simulink model "cantoni_combined_matrices"  (R2019a)
settings: Solver=FixedStepDiscrete  StartTime=0.0  StopTime=1400  FixedStep=h  RelTol=1e-3
values from neighbouring files (symbols this model uses):
  comb_contr = ss(Ac, Bc, Cc, Dc, h)    [cantoni_LMI.m]
  comb_plant_disc = c2d(comb_plant_cont,h,'zoh')    [cantoni_LMI.m]
  h = 1    [cantoni_LMI.m]    (also in distributed_workspace.mat; model_hil.m = 0.00208333333333)
settings Model: Creator=Jacob  LastModifiedBy=Jacob

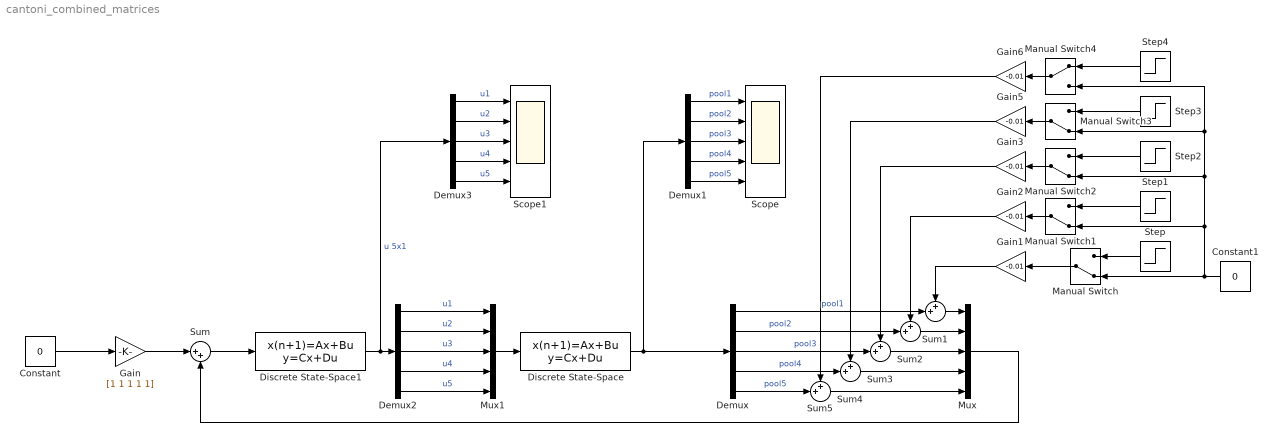
== system cantoni_combined_matrices ==
  Constant : Constant  Value=0
  Constant1 : Constant  Value=0
  Demux{,1..3} (4 alike) : Demux  Outputs=5
  Discrete State-Space : DiscreteStateSpace  A=comb_plant_disc.A  B=comb_plant_disc.B  C=comb_plant_disc.C  D=comb_plant_disc.D  SampleTime=h
  Discrete State-Space1 : DiscreteStateSpace  A=comb_contr.A  B=comb_contr.B  C=comb_contr.C  D=comb_contr.D  SampleTime=h
  Gain : Gain  Gain=[1 1 1 1 1]
  Gain{1..3,5..6} (5 alike) : Gain  Gain=-0.01
  Manual Switch{,1..3} (4 alike) : ManualSwitch  CurrentSetting=0
  Manual Switch4 : ManualSwitch
  Mux : Mux  Inputs=5
  Mux1 : Mux  Inputs=5
  Scope : Scope  NumInputPorts=5
  Scope1 : Scope  NumInputPorts=5
  Step{,1..4} (5 alike) : Step  Time=50  SampleTime=0
  Sum : Sum  Inputs=|++
  Sum{1..5} (5 alike) : Sum  Inputs=++|
  wires:
  Sum/1 -> Discrete State-Space1/1
  Discrete State-Space/1 -> Demux/1, Demux1/1
  Constant/1 -> Gain/1
  Gain/1 -> Sum/1
  Mux/1 -> Sum/2
  Demux1/1 -> Scope/1  "pool1"
  Demux1/2 -> Scope/2  "pool2"
  Demux1/3 -> Scope/3  "pool3"
  Demux1/4 -> Scope/4  "pool4"
  Demux1/5 -> Scope/5  "pool5"
  Step/1 -> Manual Switch/1
  Sum1/1 -> Mux/1
  Demux/2 -> Sum2/2  "pool2"
  Sum2/1 -> Mux/2
  Gain2/1 -> Sum2/1
  Step1/1 -> Manual Switch1/1
  Gain1/1 -> Sum1/1
  Manual Switch/1 -> Gain1/1
  Constant1/1 -> Manual Switch1/2, Manual Switch4/2, Manual Switch3/2, Manual Switch2/2, Manual Switch/2
  Manual Switch1/1 -> Gain2/1
  Demux/3 -> Sum3/2  "pool3"
  Sum3/1 -> Mux/3
  Manual Switch2/1 -> Gain3/1
  Step2/1 -> Manual Switch2/1
  Gain3/1 -> Sum3/1
  Demux/1 -> Sum1/2  "pool1"
  Demux/4 -> Sum4/2  "pool4"
  Sum4/1 -> Mux/4
  Demux/5 -> Sum5/2  "pool5"
  Sum5/1 -> Mux/5
  Step3/1 -> Manual Switch3/1
  Manual Switch3/1 -> Gain5/1
  Gain5/1 -> Sum4/1
  Manual Switch4/1 -> Gain6/1
  Step4/1 -> Manual Switch4/1
  Gain6/1 -> Sum5/1
  Discrete State-Space1/1 -> Demux3/1, Demux2/1  "u 5x1"
  Mux1/1 -> Discrete State-Space/1
  Demux2/4 -> Mux1/4  "u4"
  Demux2/3 -> Mux1/3  "u3"
  Demux2/2 -> Mux1/2  "u2"
  Demux2/1 -> Mux1/1  "u1"
  Demux2/5 -> Mux1/5  "u5"
  Demux3/5 -> Scope1/5  "u5"
  Demux3/4 -> Scope1/4  "u4"
  Demux3/3 -> Scope1/3  "u3"
  Demux3/2 -> Scope1/2  "u2"
  Demux3/1 -> Scope1/1  "u1"
